simulink model "uncontrolled"  (R2020b)
settings: Solver=VariableStepAuto  StartTime=0.0  StopTime=3*5000  RelTol=1e-8
values from neighbouring files (symbols this model uses):
  sensors = struct()    [setup.m]
  spacecraft = struct()    [setup.m]
  surfaces = struct()    [setup.m]
undefined symbols (not defined in the file or in its folder): constants, orbit
libraries: vrlib x5, library x2
settings Model: SimulationMode=accelerator  Creator=loren  LastModifiedBy=loren

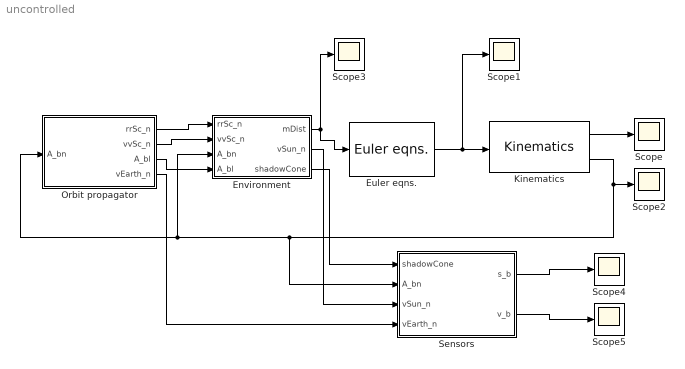
== system uncontrolled ==
  Environment : Subsystem  AncestorBlock=library/Environment
  Euler eqns. : library/Euler eqns.  SystemSampleTime=-1  VariantActivationTime=update diagram  Latency=0  AutoFrameSizeCalculation=off
  Kinematics : library/Kinematics  SystemSampleTime=-1  VariantActivationTime=update diagram  Latency=0  AutoFrameSizeCalculation=off
  Orbit propagator : Subsystem  AncestorBlock=library/Orbit propagator
  Scope{,1..5} (6 alike) : Scope
  Sensors : Subsystem  AncestorBlock=library/Sensors
  wires:
  Environment/1(mDist) -> Euler eqns./1, Scope3/1
  Euler eqns./1 -> Scope1/1, Kinematics/1
  Orbit propagator/3(A_bl) -> Environment/4(A_bl)
  Orbit propagator/2(vvSc_n) -> Environment/2(vvSc_n)
  Orbit propagator/1(rrSc_n) -> Environment/1(rrSc_n)
  Kinematics/2 -> Sensors/2(A_bn), Environment/3(A_bn), Orbit propagator/1(A_bn), Scope2/1
  Kinematics/1 -> Scope/1
  Environment/3(shadowCone) -> Sensors/1(shadowCone)
  Environment/2(vSun_n) -> Sensors/3(vSun_n)
  Sensors/1(s_b) -> Scope4/1
  Sensors/2(v_b) -> Scope5/1
  Orbit propagator/4(vEarth_n) -> Sensors/4(vEarth_n)

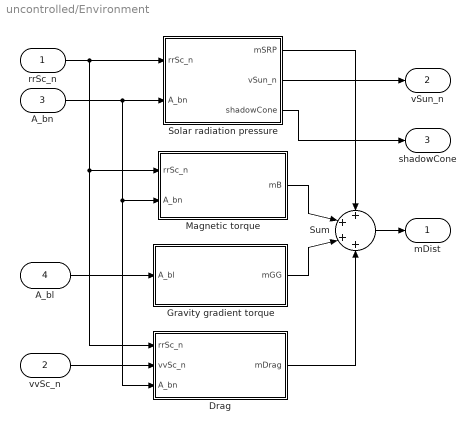
== system uncontrolled/Environment ==
  rrSc_n : Inport
  vvSc_n : Inport  Port=2
  A_bn : Inport  Port=3
  A_bl : Inport  Port=4
  Drag : Subsystem
  Gravity gradient torque : Subsystem
  Magnetic torque : Subsystem
  Solar radiation pressure : Subsystem
  Sum : Sum  Inputs=++++
  mDist : Outport
  vSun_n : Outport  Port=2
  shadowCone : Outport  Port=3
  wires:
  Solar radiation pressure/2(vSun_n) -> vSun_n/1
  A_bl/1 -> Gravity gradient torque/1(A_bl)
  Sum/1 -> mDist/1
  Magnetic torque/1(mB) -> Sum/2
  Drag/1(mDrag) -> Sum/4
  Gravity gradient torque/1(mGG) -> Sum/3
  rrSc_n/1 -> Solar radiation pressure/1(rrSc_n), Magnetic torque/1(rrSc_n), Drag/1(rrSc_n)
  vvSc_n/1 -> Drag/2(vvSc_n)
  A_bn/1 -> Solar radiation pressure/2(A_bn), Magnetic torque/2(A_bn), Drag/3(A_bn)
  Solar radiation pressure/1(mSRP) -> Sum/1
  Solar radiation pressure/3(shadowCone) -> shadowCone/1

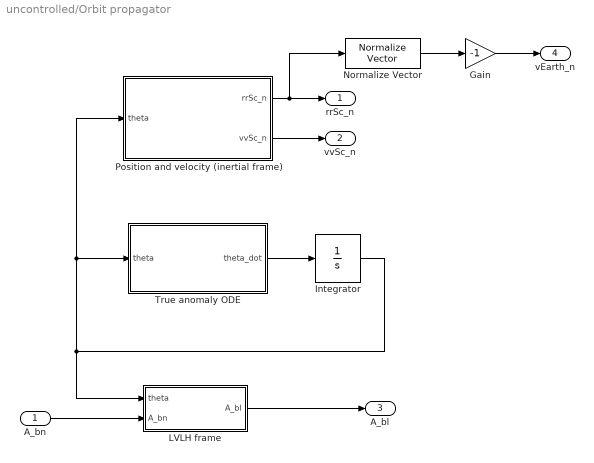
== system uncontrolled/Orbit propagator ==
  A_bn : Inport
  Gain : Gain  Gain=-1
  Integrator : Integrator  InitialCondition=orbit.theta0
  LVLH frame : Subsystem
  Normalize Vector : vrlib/Utilities/Normalize Vector  maxzero=0
  Position and velocity (inertial frame) : Subsystem
  True anomaly ODE : Subsystem
  rrSc_n : Outport
  vvSc_n : Outport  Port=2
  A_bl : Outport  Port=3
  vEarth_n : Outport  Port=4
  wires:
  A_bn/1 -> LVLH frame/2(A_bn)
  LVLH frame/1(A_bl) -> A_bl/1
  Position and velocity (inertial frame)/2(vvSc_n) -> vvSc_n/1
  Position and velocity (inertial frame)/1(rrSc_n) -> Normalize Vector/1, rrSc_n/1
  Integrator/1 -> LVLH frame/1(theta), Position and velocity (inertial frame)/1(theta), True anomaly ODE/1(theta)
  True anomaly ODE/1(theta_dot) -> Integrator/1
  Normalize Vector/1 -> Gain/1
  Gain/1 -> vEarth_n/1

== system uncontrolled/Sensors ==
  shadowCone : Inport
  A_bn : Inport  Port=2
  vSun_n : Inport  Port=3
  vEarth_n : Inport  Port=4
  Eclipse (S.T + E.H sensors) : Subsystem  TreatAsAtomicUnit=on
  Merge : Merge  InputPortOffsets=[sensors.st.nStars, sensors.st.nStars]
  Merge1 : Merge  InputPortOffsets=[sensors.st.nStars, sensors.st.nStars]
  Sunlight (S.S + E.H sensors) : Subsystem  TreatAsAtomicUnit=on
  s_b : Outport
  v_b : Outport  Port=2
  wires:
  Merge1/1 -> v_b/1
  Merge/1 -> s_b/1
  Sunlight (S.S + E.H sensors)/2(v_n) -> Merge1/2
  Eclipse (S.T + E.H sensors)/2(v_b) -> Merge1/1
  Eclipse (S.T + E.H sensors)/1(s_b) -> Merge/1
  Sunlight (S.S + E.H sensors)/1(s_b) -> Merge/2
  vEarth_n/1 -> Eclipse (S.T + E.H sensors)/2(vEarth_n), Sunlight (S.S + E.H sensors)/3(vEarth_n)
  vSun_n/1 -> Sunlight (S.S + E.H sensors)/2(vSun_n)
  A_bn/1 -> Sunlight (S.S + E.H sensors)/1(A_bn), Eclipse (S.T + E.H sensors)/1(A_bn)
  shadowCone/1 -> Sunlight (S.S + E.H sensors)/Enable, Eclipse (S.T + E.H sensors)/Enable

== system uncontrolled/Environment/Drag ==
  rrSc_n : Inport
  vvSc_n : Inport  Port=2
  A_bn : Inport  Port=3
  Constant : Constant  Value=constants.rho
  Constant1 : Constant  Value=surfaces.cd
  Constant3 : Constant  Value=surfaces.rSurf
  Constant4 : Constant  Value=surfaces.n
  Constant5 : Constant  Value=surfaces.A
  MATLAB Function : MATLAB Function  TreatAsAtomicUnit=on
  mDrag : Outport
  wires:
  Constant4/1 -> MATLAB Function/5(n)
  Constant5/1 -> MATLAB Function/6(A)
  Constant3/1 -> MATLAB Function/4(rSurf)
  Constant/1 -> MATLAB Function/7(rho)
  Constant1/1 -> MATLAB Function/8(cd)
  A_bn/1 -> MATLAB Function/3(A_bn)
  vvSc_n/1 -> MATLAB Function/2(vvSc_n)
  MATLAB Function/1(mDrag) -> mDrag/1
  rrSc_n/1 -> MATLAB Function/1(rrSc_n)

== system uncontrolled/Environment/Gravity gradient torque ==
  A_bl : Inport
  Constant : Constant  Value=[1 0 0]
  Constant1 : Constant  Value=spacecraft.I
  MATLAB Function : MATLAB Function  TreatAsAtomicUnit=on
  MatrixMultiply : Product  Multiplication=Matrix(*)
  mGG : Outport
  wires:
  A_bl/1 -> MatrixMultiply/1
  MATLAB Function/1(Mgg) -> mGG/1
  MatrixMultiply/1 -> MATLAB Function/2(c)  "c"
  Constant/1 -> MatrixMultiply/2
  Constant1/1 -> MATLAB Function/1(I)

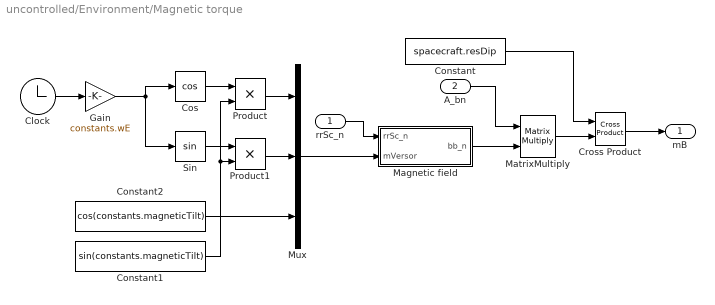
== system uncontrolled/Environment/Magnetic torque ==
  rrSc_n : Inport
  A_bn : Inport  Port=2
  Clock : Clock
  Constant : Constant  Value=spacecraft.resDip
  Constant1 : Constant  Value=sin(constants.magneticTilt)
  Constant2 : Constant  Value=cos(constants.magneticTilt)
  Cos : Trigonometry  Operator=cos
  Cross Product : vrlib/Utilities/Cross Product
  Gain : Gain  Gain=constants.wE
  Magnetic field : Subsystem
  MatrixMultiply : Product  Multiplication=Matrix(*)
  Mux : Mux  Inputs=3
  Product : Product
  Product1 : Product
  Sin : Trigonometry
  mB : Outport
  wires:
  Cross Product/1 -> mB/1
  MatrixMultiply/1 -> Cross Product/2
  Magnetic field/1(bb_n) -> MatrixMultiply/2
  Mux/1 -> Magnetic field/2(mVersor)
  rrSc_n/1 -> Magnetic field/1(rrSc_n)
  A_bn/1 -> MatrixMultiply/1
  Constant1/1 -> Product1/2, Product/2
  Product1/1 -> Mux/2
  Product/1 -> Mux/1
  Cos/1 -> Product/1
  Sin/1 -> Product1/1
  Constant2/1 -> Mux/3
  Gain/1 -> Cos/1, Sin/1
  Constant/1 -> Cross Product/1
  Clock/1 -> Gain/1

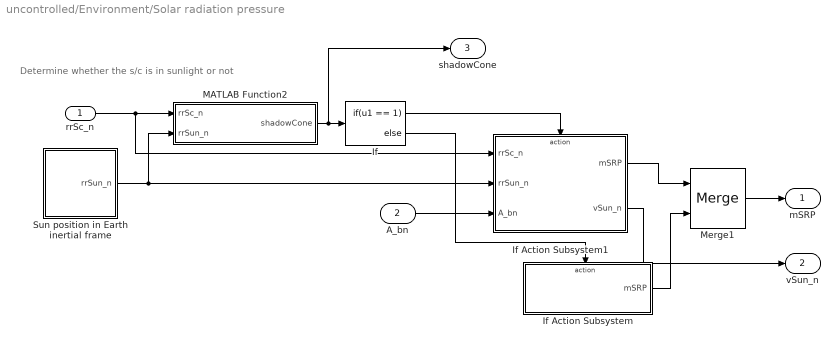
== system uncontrolled/Environment/Solar radiation pressure ==
  note: Determine whether the s/c is in sunlight or not
  rrSc_n : Inport
  A_bn : Inport  Port=2
  If : If  IfExpression=u1 == 1
  If Action Subsystem : Subsystem  TreatAsAtomicUnit=on
  If Action Subsystem1 : Subsystem  TreatAsAtomicUnit=on
  MATLAB Function2 : MATLAB Function  TreatAsAtomicUnit=on
  Merge1 : Merge
  Sun position in Earth inertial frame : Subsystem
  mSRP : Outport
  vSun_n : Outport  Port=2
  shadowCone : Outport  Port=3
  wires:
  If Action Subsystem1/2(vSun_n) -> vSun_n/1
  Sun position in Earth inertial frame/1(rrSun_n) -> MATLAB Function2/2(rrSun_n), If Action Subsystem1/2(rrSun_n)
  A_bn/1 -> If Action Subsystem1/3(A_bn)
  If Action Subsystem1/1(mSRP) -> Merge1/1
  Merge1/1 -> mSRP/1
  rrSc_n/1 -> MATLAB Function2/1(rrSc_n), If Action Subsystem1/1(rrSc_n)
  If Action Subsystem/1(mSRP) -> Merge1/2
  If/1 -> If Action Subsystem1/Action
  If/2 -> If Action Subsystem/Action
  MATLAB Function2/1(shadowCone) -> If/1, shadowCone/1

== system uncontrolled/Orbit propagator/LVLH frame ==
  theta : Inport
  A_bn : Inport  Port=2
  LVLH to inclined orbit frame : Subsystem
  Product : Product  Multiplication=Matrix(*)
  Product1 : Product  Multiplication=Matrix(*)
  R1(i) : Constant  Value=[1 0 0; 0 cos(orbit.i) sin(orbit.i); 0 -sin(orbit.i) cos(orbit.i)];
  Transpose : Math  Operator=transpose  SaturateOnIntegerOverflow=on
  A_bl : Outport
  wires:
  LVLH to inclined orbit frame/1(A_li) -> Product/1
  theta/1 -> LVLH to inclined orbit frame/1(theta)
  R1(i)/1 -> Product/2
  Product1/1 -> A_bl/1  "A_bl"
  A_bn/1 -> Product1/1
  Product/1 -> Transpose/1
  Transpose/1 -> Product1/2  "A_nl"

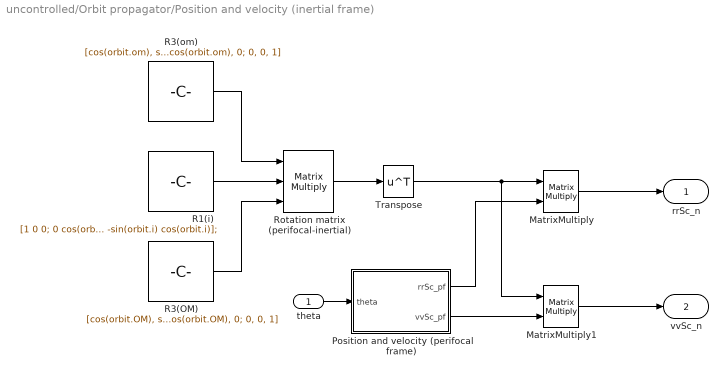
== system uncontrolled/Orbit propagator/Position and velocity (inertial frame) ==
  theta : Inport
  MatrixMultiply : Product  Multiplication=Matrix(*)
  MatrixMultiply1 : Product  Multiplication=Matrix(*)
  Position and velocity (perifocal frame) : Subsystem
  R1(i) : Constant  Value=[1 0 0; 0 cos(orbit.i) sin(orbit.i); 0 -sin(orbit.i) cos(orbit.i)];
  R3(OM) : Constant  Value=[cos(orbit.OM), sin(orbit.OM), 0; -sin(orbit.OM), cos(orbit.OM), 0; 0, 0, 1]
  R3(om) : Constant  Value=[cos(orbit.om), sin(orbit.om), 0; -sin(orbit.om), cos(orbit.om), 0; 0, 0, 1]
  Rotation matrix (perifocal-inertial) : Product  Inputs=3  Multiplication=Matrix(*)
  Transpose : Math  Operator=transpose  SaturateOnIntegerOverflow=on
  rrSc_n : Outport
  vvSc_n : Outport  Port=2
  wires:
  theta/1 -> Position and velocity (perifocal frame)/1(theta)
  Position and velocity (perifocal frame)/1(rrSc_pf) -> MatrixMultiply/2
  R3(OM)/1 -> Rotation matrix (perifocal-inertial)/3
  Transpose/1 -> MatrixMultiply/1, MatrixMultiply1/1
  Rotation matrix (perifocal-inertial)/1 -> Transpose/1
  R1(i)/1 -> Rotation matrix (perifocal-inertial)/2
  R3(om)/1 -> Rotation matrix (perifocal-inertial)/1
  MatrixMultiply1/1 -> vvSc_n/1
  Position and velocity (perifocal frame)/2(vvSc_pf) -> MatrixMultiply1/2
  MatrixMultiply/1 -> rrSc_n/1

== system uncontrolled/Orbit propagator/True anomaly ODE ==
  theta : Inport
  Add : Sum
  Constant1 : Constant
  Cos : Trigonometry  Operator=cos
  Gain : Gain  Gain=sqrt(constants.mu/orbit.a^3)
  Gain1 : Gain  Gain=(1 - orbit.e^2)^(-3/2)
  Gain2 : Gain  Gain=orbit.e
  Power : Math  Operator=square  SaturateOnIntegerOverflow=on
  theta_dot : Outport
  wires:
  Gain1/1 -> theta_dot/1
  Gain/1 -> Gain1/1
  Power/1 -> Gain/1
  Add/1 -> Power/1
  Gain2/1 -> Add/2
  Cos/1 -> Gain2/1
  Constant1/1 -> Add/1
  theta/1 -> Cos/1

== system uncontrolled/Sensors/Eclipse (S.T + E.H sensors) ==
  A_bn : Inport
  vEarth_n : Inport  Port=2
  Enable : EnablePort
  Earth-horizon sensor : Subsystem
  Matrix Concatenate : Concatenate  Mode=Multidimensional array  ConcatenateDimension=2
  Matrix Concatenate1 : Concatenate  Mode=Multidimensional array  ConcatenateDimension=2
  Star tracker : Subsystem
  s_b : Outport
  v_b : Outport  Port=2
  wires:
  Star tracker/2(vStars_n) -> Matrix Concatenate1/2
  Star tracker/1(sStars_b) -> Matrix Concatenate/2
  vEarth_n/1 -> Matrix Concatenate1/1, Earth-horizon sensor/2(vEarth_n)
  A_bn/1 -> Earth-horizon sensor/1(A_bn), Star tracker/1(A_bn)
  Earth-horizon sensor/1(vEarth_b) -> Matrix Concatenate/1
  Matrix Concatenate/1 -> s_b/1
  Matrix Concatenate1/1 -> v_b/1

== system uncontrolled/Sensors/Sunlight (S.S + E.H sensors) ==
  A_bn : Inport
  vSun_n : Inport  Port=2
  vEarth_n : Inport  Port=3
  Enable : EnablePort
  Earth-horizon sensor : Subsystem
  Sun sensor : Subsystem
  Vector Concatenate : Concatenate  Mode=Multidimensional array  ConcatenateDimension=2
  Vector Concatenate1 : Concatenate  Mode=Multidimensional array  ConcatenateDimension=2
  s_b : Outport
  v_n : Outport  Port=2
  wires:
  Vector Concatenate1/1 -> v_n/1
  Vector Concatenate/1 -> s_b/1
  Earth-horizon sensor/1(vEarth_b) -> Vector Concatenate/2
  Sun sensor/1(vSun_b) -> Vector Concatenate/1
  vSun_n/1 -> Sun sensor/2(vSun_n), Vector Concatenate1/1
  A_bn/1 -> Sun sensor/1(A_bn), Earth-horizon sensor/1(A_bn)
  vEarth_n/1 -> Vector Concatenate1/2, Earth-horizon sensor/2(vEarth_n)

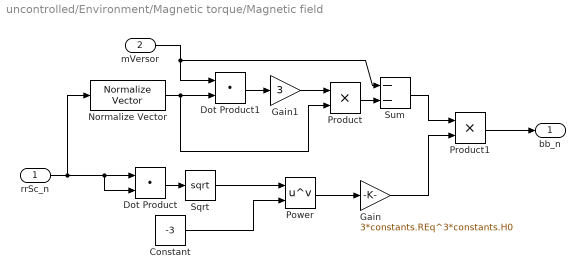
== system uncontrolled/Environment/Magnetic torque/Magnetic field ==
  rrSc_n : Inport
  mVersor : Inport  Port=2
  Constant : Constant  Value=-3
  Dot Product : DotProduct  InputSameDT=on  OutDataTypeStr=Inherit: Inherit via internal rule
  Dot Product1 : DotProduct  InputSameDT=on  OutDataTypeStr=Inherit: Inherit via internal rule
  Gain : Gain  Gain=3*constants.REq^3*constants.H0
  Gain1 : Gain  Gain=3
  Normalize Vector : vrlib/Utilities/Normalize Vector  maxzero=0
  Power : Math  Operator=pow  SaturateOnIntegerOverflow=on
  Product : Product
  Product1 : Product
  Sqrt : Sqrt  SaturateOnIntegerOverflow=on
  Sum : Sum  Inputs=--
  bb_n : Outport
  wires:
  Product1/1 -> bb_n/1
  Gain/1 -> Product1/2
  Sum/1 -> Product1/1
  Product/1 -> Sum/2
  Gain1/1 -> Product/1
  Dot Product1/1 -> Gain1/1
  mVersor/1 -> Dot Product1/1, Sum/1
  Normalize Vector/1 -> Dot Product1/2, Product/2
  Power/1 -> Gain/1
  Sqrt/1 -> Power/1
  Dot Product/1 -> Sqrt/1
  Constant/1 -> Power/2
  rrSc_n/1 -> Dot Product/1, Dot Product/2, Normalize Vector/1

== system uncontrolled/Environment/Solar radiation pressure/If Action Subsystem ==
  Action Port : ActionPort  ActionPortLabel=else
  Constant1 : Constant  Value=[0;0;0]
  mSRP : Outport
  wires:
  Constant1/1 -> mSRP/1

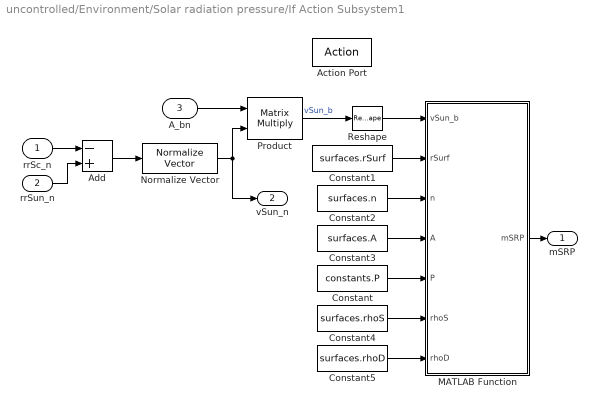
== system uncontrolled/Environment/Solar radiation pressure/If Action Subsystem1 ==
  rrSc_n : Inport
  rrSun_n : Inport  Port=2
  A_bn : Inport  Port=3
  Action Port : ActionPort  ActionPortLabel=if(u1 == 1)
  Add : Sum  Inputs=-+
  Constant : Constant  Value=constants.P
  Constant1 : Constant  Value=surfaces.rSurf
  Constant2 : Constant  Value=surfaces.n
  Constant3 : Constant  Value=surfaces.A
  Constant4 : Constant  Value=surfaces.rhoS
  Constant5 : Constant  Value=surfaces.rhoD
  MATLAB Function : MATLAB Function  TreatAsAtomicUnit=on
  Normalize Vector : vrlib/Utilities/Normalize Vector  maxzero=0
  Product : Product  Multiplication=Matrix(*)
  Reshape : Reshape  OutputDimensionality=Column vector (2-D)
  mSRP : Outport
  vSun_n : Outport  Port=2
  wires:
  Reshape/1 -> MATLAB Function/1(vSun_b)
  Constant4/1 -> MATLAB Function/6(rhoS)
  Constant5/1 -> MATLAB Function/7(rhoD)
  Constant3/1 -> MATLAB Function/4(A)
  Constant2/1 -> MATLAB Function/3(n)
  Constant1/1 -> MATLAB Function/2(rSurf)
  Constant/1 -> MATLAB Function/5(P)
  rrSc_n/1 -> Add/1
  MATLAB Function/1(mSRP) -> mSRP/1
  Add/1 -> Normalize Vector/1
  Normalize Vector/1 -> Product/2, vSun_n/1
  Product/1 -> Reshape/1  "vSun_b"
  rrSun_n/1 -> Add/2
  A_bn/1 -> Product/1

== system uncontrolled/Environment/Solar radiation pressure/Sun position in Earth inertial frame ==
  Clock : Clock
  Cos : Trigonometry  Operator=cos
  Gain : Gain  Gain=constants.nSun
  Gain1 : Gain  Gain=cos(constants.oblAngle)
  Gain2 : Gain  Gain=sin(constants.oblAngle)
  Gain3 : Gain  Gain=1*constants.AU
  Mux : Mux  Inputs=3
  Sin1 : Trigonometry
  rrSun_n : Outport
  wires:
  Gain3/1 -> rrSun_n/1
  Cos/1 -> Mux/1
  Sin1/1 -> Gain1/1, Gain2/1
  Mux/1 -> Gain3/1
  Gain1/1 -> Mux/2
  Gain/1 -> Cos/1, Sin1/1
  Clock/1 -> Gain/1
  Gain2/1 -> Mux/3

== system uncontrolled/Orbit propagator/LVLH frame/LVLH to inclined orbit frame ==
  theta : Inport
  Constant : Constant  Value=0
  Constant1 : Constant  Value=[0 0 1]
  Cos : Trigonometry  Operator=cos
  Gain : Gain  Gain=-1
  Mux : Mux  Inputs=3
  Mux1 : Mux  Inputs=3
  Sin : Trigonometry
  Vector Concatenate : Concatenate  NumInputs=3  Mode=Multidimensional array  ConcatenateDimension=2
  A_li : Outport
  wires:
  Vector Concatenate/1 -> A_li/1
  Mux1/1 -> Vector Concatenate/2
  Constant1/1 -> Vector Concatenate/3
  Mux/1 -> Vector Concatenate/1
  Gain/1 -> Mux1/1
  Constant/1 -> Mux/3, Mux1/3
  Sin/1 -> Mux/2, Gain/1
  Cos/1 -> Mux/1, Mux1/2
  theta/1 -> Cos/1, Sin/1

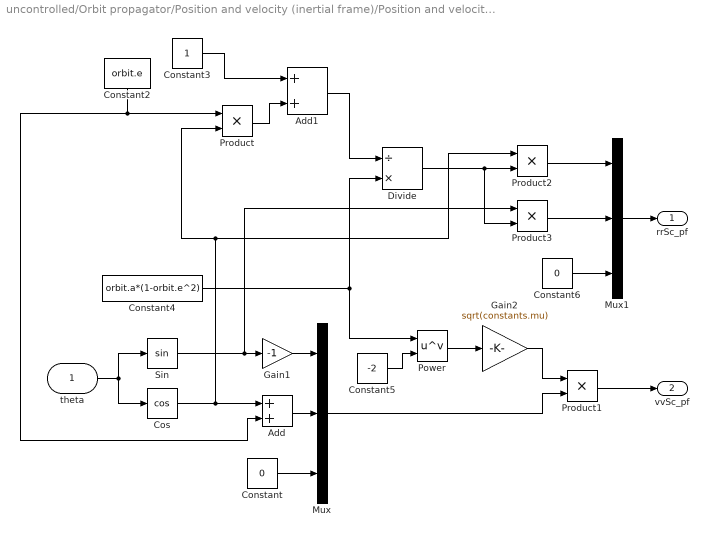
== system uncontrolled/Orbit propagator/Position and velocity (inertial frame)/Position and velocity (perifocal frame) ==
  theta : Inport
  Add : Sum
  Add1 : Sum
  Constant : Constant  Value=0
  Constant2 : Constant  Value=orbit.e
  Constant3 : Constant
  Constant4 : Constant  Value=orbit.a*(1-orbit.e^2)
  Constant5 : Constant  Value=-2
  Constant6 : Constant  Value=0
  Cos : Trigonometry  Operator=cos
  Divide : Product  Inputs=/*
  Gain1 : Gain  Gain=-1
  Gain2 : Gain  Gain=sqrt(constants.mu)
  Mux : Mux  Inputs=3
  Mux1 : Mux  Inputs=3
  Power : Math  Operator=pow  SaturateOnIntegerOverflow=on
  Product{,1..3} (4 alike) : Product
  Sin : Trigonometry
  rrSc_pf : Outport
  vvSc_pf : Outport  Port=2
  wires:
  Mux1/1 -> rrSc_pf/1
  Constant6/1 -> Mux1/3
  Product3/1 -> Mux1/2
  Product2/1 -> Mux1/1
  Divide/1 -> Product2/2, Product3/2
  Gain2/1 -> Product1/1
  Power/1 -> Gain2/1
  Constant5/1 -> Power/2
  Constant4/1 -> Power/1, Divide/2
  Add1/1 -> Divide/1
  Product/1 -> Add1/2
  Constant2/1 -> Product/1, Add/2
  Constant3/1 -> Add1/1
  Product1/1 -> vvSc_pf/1
  Constant/1 -> Mux/3
  Add/1 -> Mux/2
  Gain1/1 -> Mux/1
  Cos/1 -> Add/1, Product/2, Product2/1
  Sin/1 -> Gain1/1, Product3/1
  Mux/1 -> Product1/2
  theta/1 -> Sin/1, Cos/1

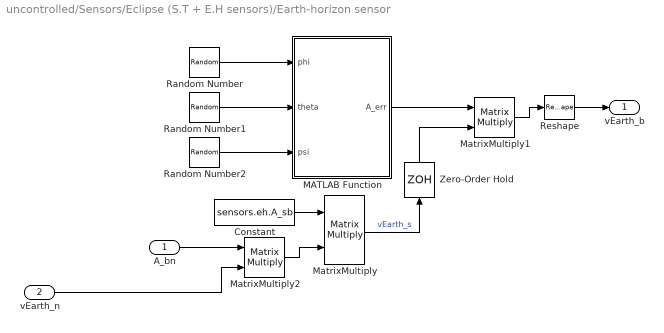
== system uncontrolled/Sensors/Eclipse (S.T + E.H sensors)/Earth-horizon sensor ==
  A_bn : Inport
  vEarth_n : Inport  Port=2
  Constant : Constant  Value=sensors.eh.A_sb
  MATLAB Function : MATLAB Function  TreatAsAtomicUnit=on
  MatrixMultiply : Product  Multiplication=Matrix(*)
  MatrixMultiply1 : Product  Multiplication=Matrix(*)
  MatrixMultiply2 : Product  Multiplication=Matrix(*)
  Random Number : RandomNumber  Variance=sensors.eh.sigmaPhi^2  Seed=randi(1e5, 1, 1)  SampleTime=max([sensors.eh.Ts, sensors.st.Ts])
  Random Number1 : RandomNumber  Variance=sensors.eh.sigmaTheta^2  Seed=randi(1e5, 1, 1)  SampleTime=max([sensors.eh.Ts, sensors.st.Ts])
  Random Number2 : RandomNumber  Variance=sensors.eh.sigmaPsi^2  Seed=randi(1e5, 1, 1)  SampleTime=max([sensors.eh.Ts, sensors.st.Ts])
  Reshape : Reshape  OutputDimensionality=Column vector (2-D)
  Zero-Order Hold : ZeroOrderHold  SampleTime=max([sensors.eh.Ts, sensors.st.Ts])
  vEarth_b : Outport
  wires:
  Zero-Order Hold/1 -> MatrixMultiply1/2
  vEarth_n/1 -> MatrixMultiply2/2
  MATLAB Function/1(A_err) -> MatrixMultiply1/1
  A_bn/1 -> MatrixMultiply2/1
  MatrixMultiply1/1 -> Reshape/1
  MatrixMultiply/1 -> Zero-Order Hold/1  "vEarth_s"
  MatrixMultiply2/1 -> MatrixMultiply/2
  Constant/1 -> MatrixMultiply/1
  Random Number/1 -> MATLAB Function/1(phi)
  Random Number1/1 -> MATLAB Function/2(theta)
  Random Number2/1 -> MATLAB Function/3(psi)
  Reshape/1 -> vEarth_b/1

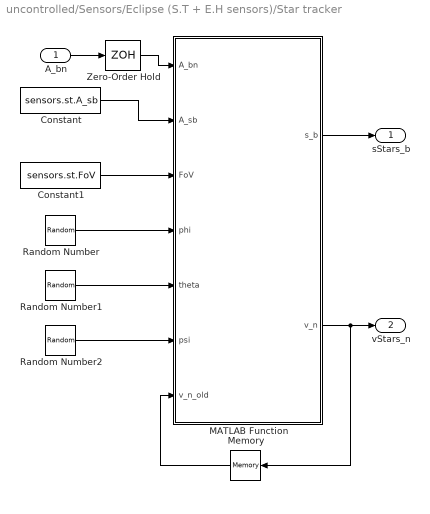
== system uncontrolled/Sensors/Eclipse (S.T + E.H sensors)/Star tracker ==
  A_bn : Inport
  Constant : Constant  Value=sensors.st.A_sb
  Constant1 : Constant  Value=sensors.st.FoV
  MATLAB Function : MATLAB Function  TreatAsAtomicUnit=on
  Memory : Memory  InitialCondition=sensors.st.vStars_n_init  InheritSampleTime=on
  Random Number : RandomNumber  Variance=sensors.st.sigmaPhi^2  Seed=randi(1e5,1,1)  SampleTime=max([sensors.eh.Ts, sensors.st.Ts])
  Random Number1 : RandomNumber  Variance=sensors.st.sigmaTheta^2  Seed=randi(1e5,1,1)  SampleTime=max([sensors.eh.Ts, sensors.st.Ts])
  Random Number2 : RandomNumber  Variance=sensors.st.sigmaPsi^2  Seed=randi(1e5,1,1)  SampleTime=max([sensors.eh.Ts, sensors.st.Ts])
  Zero-Order Hold : ZeroOrderHold  SampleTime=max([sensors.eh.Ts, sensors.st.Ts])
  sStars_b : Outport
  vStars_n : Outport  Port=2
  wires:
  Memory/1 -> MATLAB Function/7(v_n_old)
  MATLAB Function/2(v_n) -> Memory/1, vStars_n/1
  MATLAB Function/1(s_b) -> sStars_b/1
  Constant1/1 -> MATLAB Function/3(FoV)
  Zero-Order Hold/1 -> MATLAB Function/1(A_bn)
  Constant/1 -> MATLAB Function/2(A_sb)
  A_bn/1 -> Zero-Order Hold/1
  Random Number/1 -> MATLAB Function/4(phi)
  Random Number1/1 -> MATLAB Function/5(theta)
  Random Number2/1 -> MATLAB Function/6(psi)

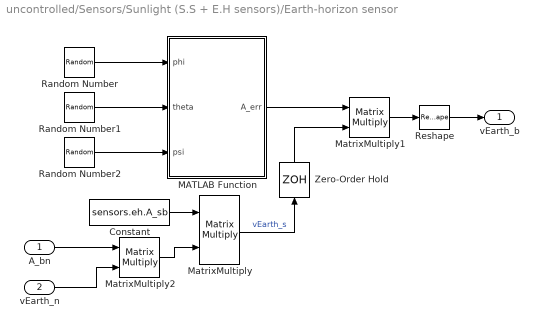
== system uncontrolled/Sensors/Sunlight (S.S + E.H sensors)/Earth-horizon sensor ==
  A_bn : Inport
  vEarth_n : Inport  Port=2
  Constant : Constant  Value=sensors.eh.A_sb
  MATLAB Function : MATLAB Function  TreatAsAtomicUnit=on
  MatrixMultiply : Product  Multiplication=Matrix(*)
  MatrixMultiply1 : Product  Multiplication=Matrix(*)
  MatrixMultiply2 : Product  Multiplication=Matrix(*)
  Random Number : RandomNumber  Variance=sensors.eh.sigmaPhi^2  Seed=randi(1e5, 1, 1)  SampleTime=max([sensors.ss.Ts, sensors.eh.Ts])
  Random Number1 : RandomNumber  Variance=sensors.eh.sigmaTheta^2  Seed=randi(1e5, 1, 1)  SampleTime=max([sensors.ss.Ts, sensors.eh.Ts])
  Random Number2 : RandomNumber  Variance=sensors.eh.sigmaPsi^2  Seed=randi(1e5, 1, 1)  SampleTime=max([sensors.ss.Ts, sensors.eh.Ts])
  Reshape : Reshape  OutputDimensionality=Column vector (2-D)
  Zero-Order Hold : ZeroOrderHold  SampleTime=max([sensors.ss.Ts, sensors.eh.Ts])
  vEarth_b : Outport
  wires:
  Zero-Order Hold/1 -> MatrixMultiply1/2
  vEarth_n/1 -> MatrixMultiply2/2
  MATLAB Function/1(A_err) -> MatrixMultiply1/1
  A_bn/1 -> MatrixMultiply2/1
  MatrixMultiply1/1 -> Reshape/1
  MatrixMultiply/1 -> Zero-Order Hold/1  "vEarth_s"
  MatrixMultiply2/1 -> MatrixMultiply/2
  Constant/1 -> MatrixMultiply/1
  Random Number/1 -> MATLAB Function/1(phi)
  Random Number1/1 -> MATLAB Function/2(theta)
  Random Number2/1 -> MATLAB Function/3(psi)
  Reshape/1 -> vEarth_b/1

== system uncontrolled/Sensors/Sunlight (S.S + E.H sensors)/Sun sensor ==
  A_bn : Inport
  vSun_n : Inport  Port=2
  Constant : Constant  Value=sensors.ss.A_sb
  If Action Subsystem : Subsystem  TreatAsAtomicUnit=on
  MatrixMultiply : Product  Multiplication=Matrix(*)
  MatrixMultiply2 : Product  Multiplication=Matrix(*)
  Measured Sun position : Subsystem  TreatAsAtomicUnit=on
  Merge : Merge
  Sensor FoV : Subsystem
  Zero-Order Hold : ZeroOrderHold  SampleTime=max([sensors.ss.Ts, sensors.eh.Ts])
  vSun_b : Outport
  wires:
  Zero-Order Hold/1 -> Measured Sun position/1(vSun_s)
  If Action Subsystem/1(vSun_b) -> Merge/2
  Merge/1 -> vSun_b/1
  Measured Sun position/1(vSun_b) -> Merge/1
  Sensor FoV/1(SunInFoV) -> If Action Subsystem/Enable, Measured Sun position/Enable
  MatrixMultiply2/1 -> MatrixMultiply/2, Sensor FoV/2(vSun_b)
  vSun_n/1 -> MatrixMultiply2/2
  Constant/1 -> Sensor FoV/1(A_sb), MatrixMultiply/1
  MatrixMultiply/1 -> Zero-Order Hold/1  "vSun_s"
  A_bn/1 -> MatrixMultiply2/1

== system uncontrolled/Sensors/Sunlight (S.S + E.H sensors)/Sun sensor/If Action Subsystem ==
  Enable : EnablePort
  Constant : Constant  Value=[NaN; NaN; NaN]
  vSun_b : Outport
  wires:
  Constant/1 -> vSun_b/1

== system uncontrolled/Sensors/Sunlight (S.S + E.H sensors)/Sun sensor/Measured Sun position ==
  vSun_s : Inport
  Enable : EnablePort
  MATLAB Function : MATLAB Function  TreatAsAtomicUnit=on
  MatrixMultiply1 : Product  Multiplication=Matrix(*)
  Random Number : RandomNumber  Variance=sensors.ss.sigmaPhi^2  Seed=randi(1e5, 1, 1)  SampleTime=max([sensors.ss.Ts, sensors.eh.Ts])
  Random Number1 : RandomNumber  Variance=sensors.ss.sigmaTheta^2  Seed=randi(1e5, 1, 1)  SampleTime=max([sensors.ss.Ts, sensors.eh.Ts])
  Random Number2 : RandomNumber  Variance=sensors.ss.sigmaPsi^2  Seed=randi(1e5, 1, 1)  SampleTime=max([sensors.ss.Ts, sensors.eh.Ts])
  vSun_b : Outport
  wires:
  vSun_s/1 -> MatrixMultiply1/2
  MATLAB Function/1(A_err) -> MatrixMultiply1/1
  MatrixMultiply1/1 -> vSun_b/1
  Random Number/1 -> MATLAB Function/1(phi)
  Random Number1/1 -> MATLAB Function/2(theta)
  Random Number2/1 -> MATLAB Function/3(psi)

== system uncontrolled/Sensors/Sunlight (S.S + E.H sensors)/Sun sensor/Sensor FoV ==
  A_sb : Inport
  vSun_b : Inport  Port=2
  Acos : Trigonometry  Operator=acos
  Constant : Constant  Value=sensors.ss.FoV
  Dot Product : DotProduct  InputSameDT=on  OutDataTypeStr=Inherit: Inherit via internal rule
  Less Than : RelationalOperator  Operator=<=  OutDataTypeStr=boolean  RndMeth=Simplest
  Normalize Vector : vrlib/Utilities/Normalize Vector  maxzero=0
  Selector : Selector  NumberOfDimensions=2  InputPortWidth=3  IndexOptions=Index vector (dialog),Index vector (dialog)  Indices=[1 2 3],[1]  OutputSizes=1,1
  SunInFoV : Outport
  wires:
  Less Than/1 -> SunInFoV/1
  Constant/1 -> Less Than/2
  Acos/1 -> Less Than/1
  Dot Product/1 -> Acos/1
  vSun_b/1 -> Dot Product/2
  Normalize Vector/1 -> Dot Product/1
  Selector/1 -> Normalize Vector/1
  A_sb/1 -> Selector/1

== matlab function uncontrolled/Sensors/Sunlight (S.S + E.H sensors)/Earth-horizon sensor/MATLAB Function ==
  data: phi input; A_err output; theta input; psi input
function A_err = error_matrix(phi, theta, psi)

A_err = [cos(psi)*cos(theta), cos(psi)*sin(theta)*sin(phi) + sin(psi)*cos(phi),...
    -cos(psi)*sin(theta)*cos(phi) + sin(psi)*sin(phi);...
    -sin(psi)*cos(theta), -sin(psi)*sin(theta)*sin(phi) + cos(psi)*cos(phi),...
    sin(psi)*sin(theta)*cos(phi) + cos(psi)*sin(phi);...
    sin(theta), -cos(theta)*sin(phi), cos(theta)*cos(phi)];
            
end

== matlab function uncontrolled/Sensors/Sunlight (S.S + E.H sensors)/Sun sensor/Measured Sun position/MATLAB Function ==
  data: phi input; A_err output; theta input; psi input
function A_err = error_matrix(phi, theta, psi)

A_err = [cos(psi)*cos(theta), cos(psi)*sin(theta)*sin(phi) + sin(psi)*cos(phi),...
    -cos(psi)*sin(theta)*cos(phi) + sin(psi)*sin(phi);...
    -sin(psi)*cos(theta), -sin(psi)*sin(theta)*sin(phi) + cos(psi)*cos(phi),...
    sin(psi)*sin(theta)*cos(phi) + cos(psi)*sin(phi);...
    sin(theta), -cos(theta)*sin(phi), cos(theta)*cos(phi)];
            
end

== matlab function uncontrolled/Sensors/Eclipse (S.T + E.H sensors)/Earth-horizon sensor/MATLAB Function ==
  data: phi input; A_err output; theta input; psi input
function A_err = error_matrix(phi, theta, psi)

A_err = [cos(psi)*cos(theta), cos(psi)*sin(theta)*sin(phi) + sin(psi)*cos(phi),...
    -cos(psi)*sin(theta)*cos(phi) + sin(psi)*sin(phi);...
    -sin(psi)*cos(theta), -sin(psi)*sin(theta)*sin(phi) + cos(psi)*cos(phi),...
    sin(psi)*sin(theta)*cos(phi) + cos(psi)*sin(phi);...
    sin(theta), -cos(theta)*sin(phi), cos(theta)*cos(phi)];
            
end

== matlab function uncontrolled/Environment/Drag/MATLAB Function ==
  data: rrSc_n input; mDrag output; vvSc_n input; A_bn input; rSurf input; n input; A input; rho input; cd input
function  mDrag = drag(rrSc_n, vvSc_n, A_bn, rSurf, n, A, rho, cd)

wE = 7.2921150e-5; %[rad/s]
vvRel_n = [vvSc_n(1) + wE*rrSc_n(2); vvSc_n(2) - wE*rrSc_n(1); vvSc_n(3)];
vvRel_b = A_bn*vvRel_n;

vRel = norm(vvRel_n);
vRel_b = norm(vvRel_b);
vvVersor = vvRel_b/vRel_b;

c = -1/2*rho*cd*vRel^2.*vvVersor;

mDrag = zeros(3,1);

for k = 1:size(rSurf,1)
        n_dot = dot(n(:,k), vvVersor);
    if n_dot > 0
        A_cross = A(k)*n_dot;
        Fdrag_i = c*A_cross;
        mDrag = mDrag + cross(rSurf(:,k), Fdrag_i);
    end
end

end

== matlab function uncontrolled/Environment/Gravity gradient torque/MATLAB Function ==
  data: Mgg output; I input; c input
function Mgg = gravity_gradient(I, c)

mu = 398600;
REq = 6371.8e3;

c1 = c(1);
c2 = c(2);
c3 = c(3);
Ix = I(1,1);
Iy = I(2,2);
Iz = I(3,3);

Mgg = 3*mu/(REq^3)*[(Iz - Iy)*c2*c3;...
    (Ix - Iz)*c1*c3;...
    (Iy - Ix)*c1*c2];

end

== matlab function uncontrolled/Sensors/Eclipse (S.T + E.H sensors)/Star tracker/MATLAB Function ==
  data: A_bn input; s_b output; A_sb input; FoV input; phi input; theta input; psi input; v_n output; v_n_old input; sensors parameter
function [s_b, v_n] = starTracker(A_bn, A_sb, FoV, phi, theta, psi, v_n_old, sensors)

nStars = sensors.st.nStars;

A_bs = A_sb';
A_ns = A_bn'*A_bs;

s_b = zeros(3,nStars); 
v_n = zeros(3,nStars);

El = zeros(nStars,1);
Az = zeros(nStars,1);
A_err = zeros(nStars);
v_s = zeros(3,1);

for k = 0:nStars-1
    
    s_b_old = A_bn*v_n_old(:,end-k);
    v_s_old = A_sb*s_b_old;
    
    El_old = asin(v_s_old(3));
    Az_old = acos(v_s_old(1)/cos(El_old));
    
    if v_s_old(2) <= 0
        El_old = 2*pi - El_old;
    end
    
    if abs(Az_old) > FoV(1)/2 || abs(El_old) > FoV(2)/2
        Az(end-k) = 0.2*FoV(1)*(-1 + 2*rand(1,1));
        El(end-k) = 0.2*FoV(2)*(-1 + 2*rand(1,1));
        v_s = [cos(El(end-k))*cos(Az(end-k));...
            cos(El(end-k))*sin(Az(end-k));...
            sin(El(end-k))];
        A_err = [cos(psi)*cos(theta), cos(psi)*sin(theta)*sin(phi) + sin(psi)*cos(phi),...
            -cos(psi)*sin(theta)*cos(phi) + sin(psi)*sin(phi);...
            -sin(psi)*cos(theta), -sin(psi)*sin(theta)*sin(phi) + cos(psi)*cos(phi),...
            sin(psi)*sin(theta)*cos(phi) + cos(psi)*sin(phi);...
            sin(theta), -cos(theta)*sin(phi), cos(theta)*cos(phi)];
    else
        A_err = eye(3);
        v_s = v_s_old;
    end
   
   s_s = A_err*v_s;
   s_b(1:3,end-k) = A_bs*s_s; 
   v_n(1:3,end-k) = A_ns*v_s;
   
end

end

== matlab function uncontrolled/Environment/Solar radiation pressure/If Action Subsystem1/MATLAB Function ==
  data: vSun_b input; rSurf input; n input; A input; mSRP output; P input; rhoS input; rhoD input
function mSRP = srp(vSun_b, rSurf, n, A, P, rhoS, rhoD)

mSRP = zeros(3,1);

for k = 1:size(rSurf,1)
    n_b = n(:,k);
    s_dot = dot(vSun_b, n_b);
    if s_dot > 0
        rhoS_temp = rhoS(k);
        Fsrp_i = - P*A(k)*s_dot.*((1-rhoS_temp).*vSun_b +...
            (2*rhoS_temp*s_dot + 2/3*rhoD(k)).*n_b);
        mSRP = mSRP + cross(rSurf(:,k), Fsrp_i);
    end
end

% aggiungere questione su "ombra"

end

== matlab function uncontrolled/Environment/Solar radiation pressure/MATLAB Function2 ==
  data: rrSc_n input; shadowCone output; rrSun_n input
function shadowCone = cone(rrSc_n, rrSun_n)

% PROTOTYPE:
%  shadow_cone = cone(rr_sc, rr_sun_n)
% 
% DESCRIPTION:
%   This function returns a parameter that is 1 if the s/c is out of the 
%   planet's shadow cone (SRP effects considerable) or 0 if the s/c is 
%   inside the planet's shadow cone (NO SRP)
% 
% INPUT:
% rr_sc:            geocentric position vector of the s/c
% rr_sun_n:        geocentric position vector of the sun
%
% OUTPUT:
% shadow_cone:      boolean parameter (0 or 1)
%
% CONTRIBUTORS:
% Velo Giacomo
%
% VERSIONS:
% 2019-12-10 first version
%
% CALLED FUNCTIONS:
%     none


Req = 6378.1;
r = norm(rrSc_n);     
r_sun = norm(rrSun_n);
% Angle between s/c geocentric position and the tangent to Earth's surface
theta_sc = acos(Req/r);
% Angle between sun geocentric position and the tangent to Earth's surface
theta_sun = acos(Req/r_sun);
% Angle between s/c geocentric position and sun geocentric position
theta = acos(dot(rrSc_n, rrSun_n)/(r*r_sun));

% If the s/c is inside the shadow cone of the planet the value of
% shadow_cone will be = 0

    if theta_sc + theta_sun <= theta
        shadowCone = 0;
    else
        shadowCone = 1;
    end

end
